simulink model "deel1_simulink"  (R2020b)
settings: Solver=FixedStepAuto  StartTime=0.0  StopTime=100  FixedStep=1e-3  RelTol=1e-3
settings Model: Creator=Xander  LastModifiedBy=Xander
settings DataIOCC: ReturnWorkspaceOutputs=off

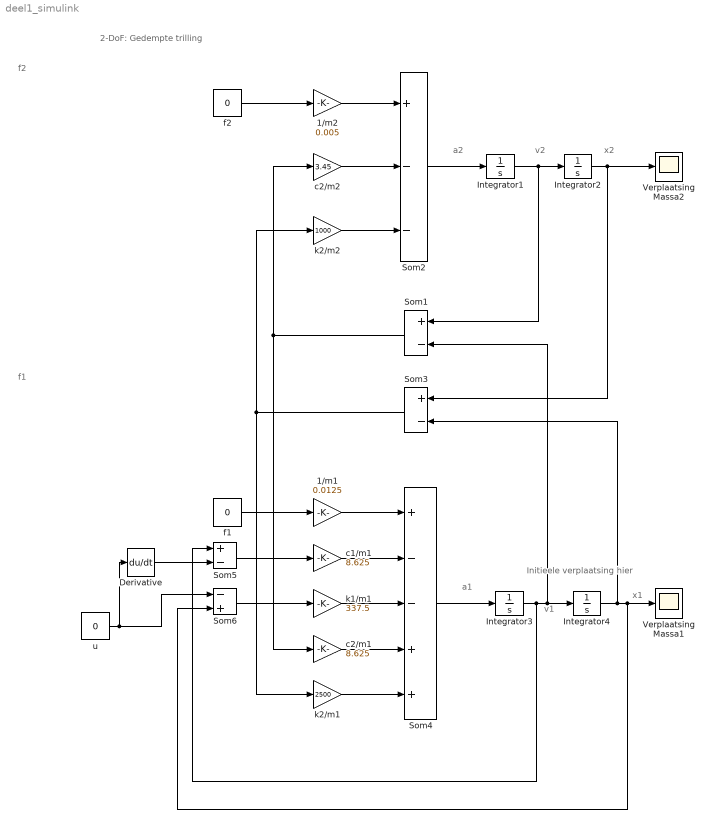
== system deel1_simulink ==
  note: f1
  note: f2
  note: x1
  note: x2
  note: Initieele verplaatsing hier
  note: 2-DoF: Gedempte trilling
  note: v2
  note: a2
  note: v1
  note: a1
  1/m1 : Gain  Gain=0.0125
  1/m2 : Gain  Gain=0.005
  Derivative : Derivative
  Integrator1 : Integrator
  Integrator2 : Integrator
  Integrator3 : Integrator
  Integrator4 : Integrator  InitialCondition=0.1
  Som1 : Sum  Inputs=+-
  Som2 : Sum  Inputs=+--
  Som3 : Sum  Inputs=+-
  Som4 : Sum  Inputs=+--++
  Som5 : Sum  Inputs=+-
  Som6 : Sum  Inputs=-+
  Verplaatsing Massa1 : Scope
  Verplaatsing Massa2 : Scope
  c1/m1 : Gain  Gain=8.625
  c2/m1 : Gain  Gain=8.625
  c2/m2 : Gain  Gain=3.45
  f1 : Constant  Value=0
  f2 : Constant  Value=0
  k1/m1 : Gain  Gain=337.5
  k2/m1 : Gain  Gain=2500
  k2/m2 : Gain  Gain=1000
  u : Constant  Value=0
  wires:
  1/m2/1 -> Som2/1
  c2/m2/1 -> Som2/2
  k2/m2/1 -> Som2/3
  Som2/1 -> Integrator1/1
  Integrator1/1 -> Som1/1, Integrator2/1
  Integrator2/1 -> Som3/1, Verplaatsing Massa2/1
  f2/1 -> 1/m2/1
  Som1/1 -> c2/m1/1, c2/m2/1
  Som3/1 -> k2/m2/1, k2/m1/1
  1/m1/1 -> Som4/1
  c1/m1/1 -> Som4/2
  k1/m1/1 -> Som4/3
  c2/m1/1 -> Som4/4
  k2/m1/1 -> Som4/5
  f1/1 -> 1/m1/1
  Som5/1 -> c1/m1/1
  Som6/1 -> k1/m1/1
  u/1 -> Derivative/1, Som6/1
  Integrator4/1 -> Som3/2, Som6/2, Verplaatsing Massa1/1
  Integrator3/1 -> Som5/1, Integrator4/1, Som1/2
  Som4/1 -> Integrator3/1
  Derivative/1 -> Som5/2
